simulink model "ADP_RPI"  (R2017a)
settings: Solver=FixedStepAuto  StartTime=0.0  StopTime=inf  RelTol=1e-3
InitFcn:
  | ADP_Init
  | RPI3_SPI_Int
values from neighbouring files (symbols this model uses):
  K = 0.5*(R_Mat_ADP^-1)*B'*P_Mat    [ADP_Init.m]
  T = 1    [ADP_Init.m]
  tau = 0.01    [ADP_Init.m]
  wcInit = weights    [ADP_Init.m]
undefined symbols (not defined in the file or in its folder): spiPeriod
libraries: simulink x4, embdlinuxlib x4, simulink_extras x2
settings Model: SimulationMode=external  ExtModeTrigDuration=10000  Creator=gjaniak  LastModifiedBy=gjaniak
settings SolverCC: PositivePriorityOrder=on
settings OptimizationCC: PassReuseOutputArgsAs=Individual arguments  MaxStackSize=64
settings DebuggingCC: ParameterTunabilityLossMsg=error
settings HardwareCC: ProdBitPerPointer=32  ProdBitPerSizeT=32  ProdBitPerPtrDiffT=32  ProdLargestAtomicInteger=Long  ProdLargestAtomicFloat=Double  ProdWordSize=32  ProdHWDeviceType=ARM Compatible->ARM Cortex
settings SFSimCC: MATLABDynamicMemAlloc=off
settings RTWCC: SystemTargetFile=ert.tlc  HardwareBoard=Raspberry Pi  TLCOptions="-aInlineSetEventsForThisBaseRateFcn=TLC_FALSE -aSuppressMultiTaskScheduler=TLC_FALSE  -aRateBasedStepFcn=0"  TemplateMakefile=ert_default_tmf  Description=Embedded Coder  GenerateReport=on  Toolchain=GNU GCC Raspberry Pi  IncludeHyperlinkInReport=on  LaunchReport=on  GenerateTraceInfo=on  GenerateTraceReport=on  GenerateTraceReportSl=on  GenerateTraceReportSf=on  GenerateTraceReportEml=on
settings CodeAppCC: ForceParamTrailComments=on  IgnoreCustomStorageClasses=off  OperatorAnnotations=on  SimulinkDataObjDesc=on  SFDataObjDesc=on  MATLABFcnDesc=on  InsertBlockDesc=on  MATLABSourceComments=on
settings ERTTargetCC: SupportContinuousTime=on  SupportVariableSizeSignals=on

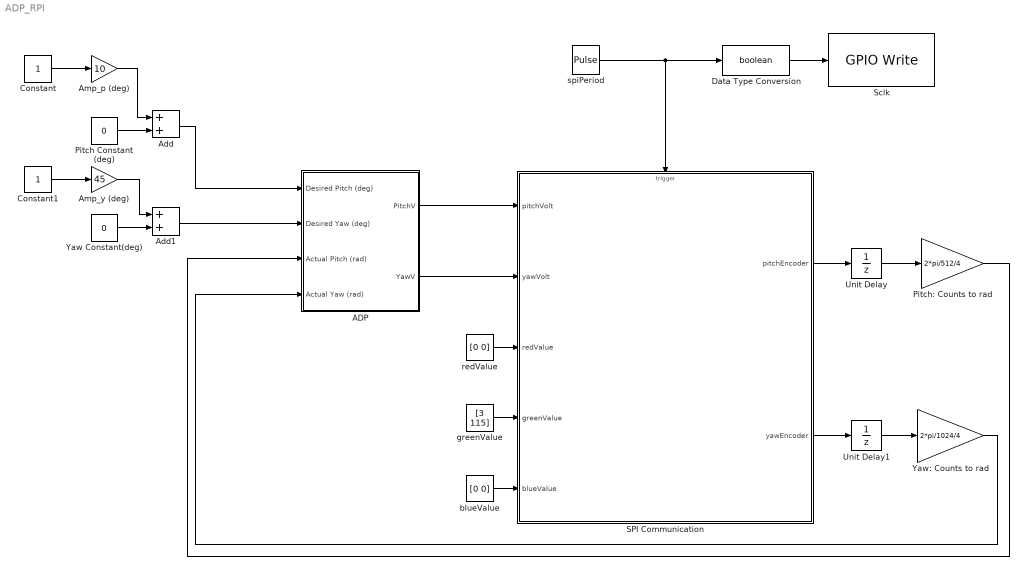
== system ADP_RPI ==
  ADP : Subsystem
  Add : Sum
  Add1 : Sum
  Amp_p (deg) : Gain  Gain=10
  Amp_y (deg) : Gain  Gain=45
  Constant : Constant
  Constant1 : Constant
  Data Type Conversion : DataTypeConversion  OutDataTypeStr=boolean
  Pitch Constant (deg) : Constant  Value=0
  Pitch: Counts to rad : Gain  Gain=2*pi/512/4
  SPI Communication : Subsystem  TreatAsAtomicUnit=on
  Sclk : embdlinuxlib/GPIO Write  board=Pi 3 Model B  gpio=11  direction=Output  blockPlatform=Raspberry Pi
  Unit Delay : UnitDelay  SampleTime=-1
  Unit Delay1 : UnitDelay  SampleTime=-1
  Yaw Constant(deg) : Constant  Value=0
  Yaw: Counts to rad : Gain  Gain=2*pi/1024/4
  blueValue : Constant  Value=[0 0]
  greenValue : Constant  Value=[3 115]
  redValue : Constant  Value=[0 0]
  spiPeriod : DiscretePulseGenerator  PulseType=Time based  Period=spiPeriod  PulseWidth=50
  wires:
  Pitch Constant (deg)/1 -> Add/2
  Amp_p (deg)/1 -> Add/1
  Yaw Constant(deg)/1 -> Add1/2
  Amp_y (deg)/1 -> Add1/1
  Constant/1 -> Amp_p (deg)/1
  Constant1/1 -> Amp_y (deg)/1
  Data Type Conversion/1 -> Sclk/1
  blueValue/1 -> SPI Communication/5(blueValue)
  Unit Delay1/1 -> Yaw: Counts to rad/1
  spiPeriod/1 -> SPI Communication/Trigger, Data Type Conversion/1
  SPI Communication/1(pitchEncoder) -> Unit Delay/1
  SPI Communication/2(yawEncoder) -> Unit Delay1/1
  greenValue/1 -> SPI Communication/4(greenValue)
  redValue/1 -> SPI Communication/3(redValue)
  Unit Delay/1 -> Pitch: Counts to rad/1
  ADP/1(PitchV) -> SPI Communication/1(pitchVolt)
  ADP/2(YawV) -> SPI Communication/2(yawVolt)
  Add/1 -> ADP/1(Desired Pitch (deg))
  Add1/1 -> ADP/2(Desired Yaw (deg))
  Yaw: Counts to rad/1 -> ADP/4(Actual Yaw (rad))
  Pitch: Counts to rad/1 -> ADP/3(Actual Pitch (rad))

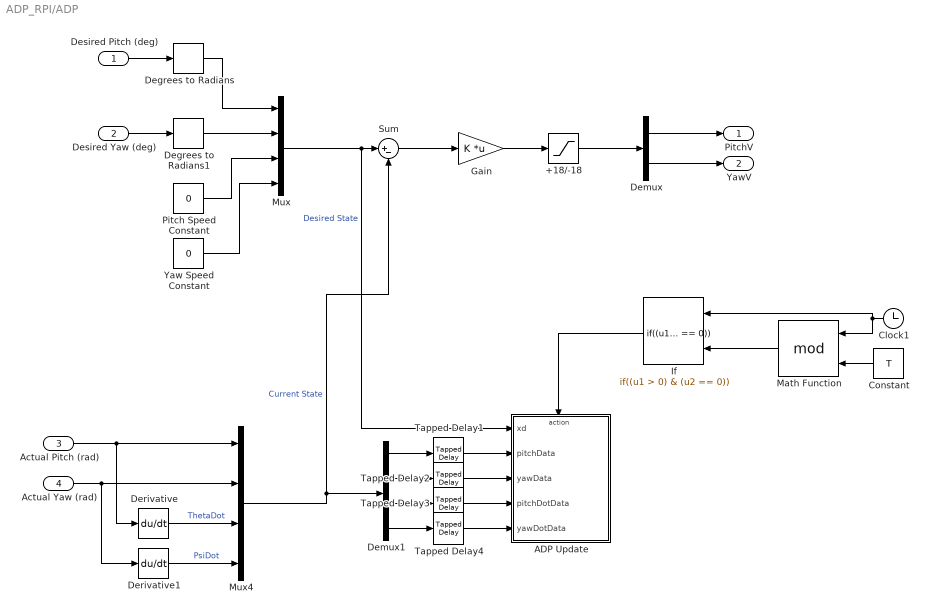
== system ADP_RPI/ADP ==
  Desired Pitch (deg) : Inport
  Desired Yaw (deg) : Inport  Port=2
  Actual Pitch (rad) : Inport  Port=3
  Actual Yaw (rad) : Inport  Port=4
  +18/-18 : Saturate  UpperLimit=18  LowerLimit=-18
  ADP Update : Subsystem  TreatAsAtomicUnit=on
  Clock1 : Clock
  Constant : Constant  Value=T
  Degrees to Radians : simulink_extras/Transformations/Degrees to Radians
  Degrees to Radians1 : simulink_extras/Transformations/Degrees to Radians
  Demux : Demux  Outputs=2
  Demux1 : Demux
  Derivative : Derivative
  Derivative1 : Derivative
  Gain : Gain  Gain=K  Multiplication=Matrix(K*u)
  If : If  NumInputs=2  IfExpression=(u1 > 0) & (u2 == 0)  ShowElse=off
  Math Function : Math  Operator=mod  SaturateOnIntegerOverflow=on
  Mux : Mux
  Mux4 : Mux
  Pitch Speed Constant : Constant  Value=0
  Sum : Sum  Inputs=|+-
  Tapped Delay{1..4} (4 alike) : simulink/Discrete/Tapped Delay  vinit=0.0  samptime=-1  NumDelays=floor(T/tau)  DelayOrder=Oldest  includeCurrent=off
  Yaw Speed Constant : Constant  Value=0
  PitchV : Outport
  YawV : Outport  Port=2
  wires:
  Sum/1 -> Gain/1
  Gain/1 -> +18/-18/1
  +18/-18/1 -> Demux/1
  Demux/1 -> PitchV/1
  Demux/2 -> YawV/1
  If/1 -> ADP Update/Action
  Math Function/1 -> If/2
  Constant/1 -> Math Function/2
  Clock1/1 -> If/1, Math Function/1
  Demux1/1 -> Tapped Delay1/1
  Tapped Delay1/1 -> ADP Update/2(pitchData)
  Demux1/2 -> Tapped Delay2/1
  Tapped Delay2/1 -> ADP Update/3(yawData)
  Demux1/3 -> Tapped Delay3/1
  Tapped Delay3/1 -> ADP Update/4(pitchDotData)
  Demux1/4 -> Tapped Delay4/1
  Tapped Delay4/1 -> ADP Update/5(yawDotData)
  Mux/1 -> ADP Update/1(xd), Sum/1  "Desired State"
  Degrees to Radians1/1 -> Mux/2
  Yaw Speed Constant/1 -> Mux/4
  Degrees to Radians/1 -> Mux/1
  Pitch Speed Constant/1 -> Mux/3
  Desired Pitch (deg)/1 -> Degrees to Radians/1
  Desired Yaw (deg)/1 -> Degrees to Radians1/1
  Actual Pitch (rad)/1 -> Mux4/1, Derivative/1
  Actual Yaw (rad)/1 -> Mux4/2, Derivative1/1
  Mux4/1 -> Sum/2, Demux1/1  "Current State"
  Derivative/1 -> Mux4/3  "ThetaDot"
  Derivative1/1 -> Mux4/4  "PsiDot"

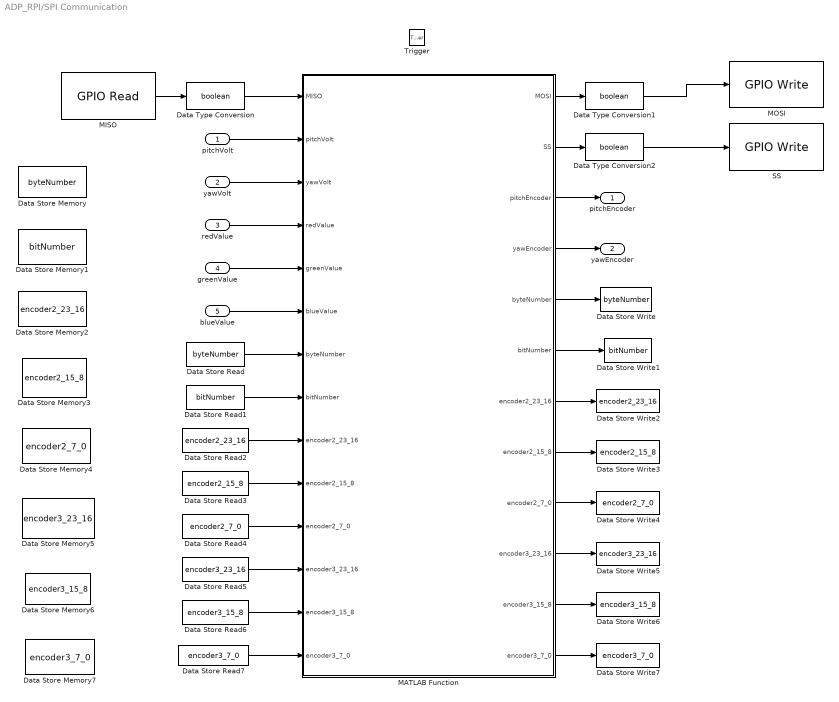
== system ADP_RPI/SPI Communication ==
  pitchVolt : Inport
  yawVolt : Inport  Port=2
  redValue : Inport  Port=3
  greenValue : Inport  Port=4
  blueValue : Inport  Port=5
  Trigger : TriggerPort  VariantControl=Variant
  Data Store Memory : DataStoreMemory  DataStoreName=byteNumber  ReadBeforeWriteMsg=warning  WriteAfterWriteMsg=warning  WriteAfterReadMsg=warning  ShowAdditionalParam=off
  Data Store Memory1 : DataStoreMemory  DataStoreName=bitNumber  ReadBeforeWriteMsg=warning  WriteAfterWriteMsg=warning  WriteAfterReadMsg=warning  ShowAdditionalParam=off
  Data Store Memory2 : DataStoreMemory  DataStoreName=encoder2_23_16  ReadBeforeWriteMsg=warning  WriteAfterWriteMsg=warning  WriteAfterReadMsg=warning  InitialValue=[0 0 0 0 0 0 0 0]  ShowAdditionalParam=off
  Data Store Memory3 : DataStoreMemory  DataStoreName=encoder2_15_8  ReadBeforeWriteMsg=warning  WriteAfterWriteMsg=warning  WriteAfterReadMsg=warning  InitialValue=[0 0 0 0 0 0 0 0]  ShowAdditionalParam=off
  Data Store Memory4 : DataStoreMemory  DataStoreName=encoder2_7_0  ReadBeforeWriteMsg=warning  WriteAfterWriteMsg=warning  WriteAfterReadMsg=warning  InitialValue=[0 0 0 0 0 0 0 0]  ShowAdditionalParam=off
  Data Store Memory5 : DataStoreMemory  DataStoreName=encoder3_23_16  ReadBeforeWriteMsg=warning  WriteAfterWriteMsg=warning  WriteAfterReadMsg=warning  InitialValue=[0 0 0 0 0 0 0 0]  ShowAdditionalParam=off
  Data Store Memory6 : DataStoreMemory  DataStoreName=encoder3_15_8  ReadBeforeWriteMsg=warning  WriteAfterWriteMsg=warning  WriteAfterReadMsg=warning  InitialValue=[0 0 0 0 0 0 0 0]  ShowAdditionalParam=off
  Data Store Memory7 : DataStoreMemory  DataStoreName=encoder3_7_0  ReadBeforeWriteMsg=warning  WriteAfterWriteMsg=warning  WriteAfterReadMsg=warning  InitialValue=[0 0 0 0 0 0 0 0]  ShowAdditionalParam=off
  Data Store Read1 : DataStoreRead  DataStoreName=bitNumber
  Data Store Read2 : DataStoreRead  DataStoreName=encoder2_23_16
  Data Store Read3 : DataStoreRead  DataStoreName=encoder2_15_8
  Data Store Read4 : DataStoreRead  DataStoreName=encoder2_7_0
  Data Store Read5 : DataStoreRead  DataStoreName=encoder3_23_16
  Data Store Read6 : DataStoreRead  DataStoreName=encoder3_15_8
  Data Store Read7 : DataStoreRead  DataStoreName=encoder3_7_0
  Data Store Write : DataStoreWrite  DataStoreName=byteNumber
  Data Store Write1 : DataStoreWrite  DataStoreName=bitNumber
  Data Store Write2 : DataStoreWrite  DataStoreName=encoder2_23_16
  Data Store Write3 : DataStoreWrite  DataStoreName=encoder2_15_8
  Data Store Write4 : DataStoreWrite  DataStoreName=encoder2_7_0
  Data Store Write5 : DataStoreWrite  DataStoreName=encoder3_23_16
  Data Store Write6 : DataStoreWrite  DataStoreName=encoder3_15_8
  Data Store Write7 : DataStoreWrite  DataStoreName=encoder3_7_0
  Data Store Read : DataStoreRead  DataStoreName=byteNumber
  Data Type Conversion : DataTypeConversion  OutDataTypeStr=boolean
  Data Type Conversion1 : DataTypeConversion  OutDataTypeStr=boolean
  Data Type Conversion2 : DataTypeConversion  OutDataTypeStr=boolean
  MATLAB Function : MATLAB Function  TreatAsAtomicUnit=on
  MISO : embdlinuxlib/GPIO Read  board=Pi 3 Model B  gpio=9  internalResistor=Off  sampleTime=inf  direction=Input  blockPlatform=Raspberry Pi
  MOSI : embdlinuxlib/GPIO Write  board=Pi 3 Model B  gpio=10  direction=Output  blockPlatform=Raspberry Pi
  "SS " : embdlinuxlib/GPIO Write  board=Pi 3 Model B  gpio=8  direction=Output  blockPlatform=Raspberry Pi
  pitchEncoder : Outport
  yawEncoder : Outport  Port=2
  wires:
  blueValue/1 -> MATLAB Function/6(blueValue)
  greenValue/1 -> MATLAB Function/5(greenValue)
  redValue/1 -> MATLAB Function/4(redValue)
  yawVolt/1 -> MATLAB Function/3(yawVolt)
  pitchVolt/1 -> MATLAB Function/2(pitchVolt)
  MATLAB Function/4(yawEncoder) -> yawEncoder/1
  MATLAB Function/3(pitchEncoder) -> pitchEncoder/1
  Data Type Conversion/1 -> MATLAB Function/1(MISO)
  MATLAB Function/1(MOSI) -> Data Type Conversion1/1
  MATLAB Function/2(SS) -> Data Type Conversion2/1
  MISO/1 -> Data Type Conversion/1
  Data Type Conversion1/1 -> MOSI/1
  Data Type Conversion2/1 -> "SS "/1
  Data Store Read/1 -> MATLAB Function/7("byteNumber ")
  Data Store Read1/1 -> MATLAB Function/8("bitNumber ")
  Data Store Read2/1 -> MATLAB Function/9("encoder2_23_16 ")
  Data Store Read3/1 -> MATLAB Function/10("encoder2_15_8 ")
  Data Store Read4/1 -> MATLAB Function/11("encoder2_7_0 ")
  Data Store Read5/1 -> MATLAB Function/12("encoder3_23_16 ")
  Data Store Read6/1 -> MATLAB Function/13("encoder3_15_8 ")
  Data Store Read7/1 -> MATLAB Function/14("encoder3_7_0 ")
  MATLAB Function/5(byteNumber) -> Data Store Write/1
  MATLAB Function/6(bitNumber) -> Data Store Write1/1
  MATLAB Function/7(encoder2_23_16) -> Data Store Write2/1
  MATLAB Function/8(encoder2_15_8) -> Data Store Write3/1
  MATLAB Function/9(encoder2_7_0) -> Data Store Write4/1
  MATLAB Function/10(encoder3_23_16) -> Data Store Write5/1
  MATLAB Function/11(encoder3_15_8) -> Data Store Write6/1
  MATLAB Function/12(encoder3_7_0) -> Data Store Write7/1

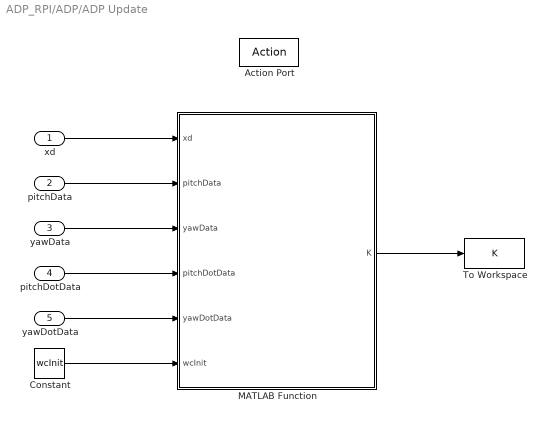
== system ADP_RPI/ADP/ADP Update ==
  xd : Inport
  pitchData : Inport  Port=2
  yawData : Inport  Port=3
  pitchDotData : Inport  Port=4
  yawDotData : Inport  Port=5
  Action Port : ActionPort  ActionType=then
  Constant : Constant  Value=wcInit
  MATLAB Function : MATLAB Function  TreatAsAtomicUnit=on
  To Workspace : ToWorkspace  VariableName=K  SampleTime=-1
  wires:
  MATLAB Function/1(K) -> To Workspace/1
  yawData/1 -> MATLAB Function/3(yawData)
  pitchDotData/1 -> MATLAB Function/4(pitchDotData)
  yawDotData/1 -> MATLAB Function/5(yawDotData)
  pitchData/1 -> MATLAB Function/2(pitchData)
  xd/1 -> MATLAB Function/1(xd)
  Constant/1 -> MATLAB Function/6(wcInit)

== matlab function ADP_RPI/SPI Communication/MATLAB Function ==
  data: MISO input; MOSI output; pitchVolt input; yawVolt input; redValue input; greenValue input; blueValue input; byteNumber input; bitNumber input; encoder2_23_16 input; encoder2_15_8 input; encoder2_7_0 input; encoder3_23_16 input; encoder3_15_8 input; encoder3_7_0 input; SS output; pitchEncoder output; yawEncoder output; byteNumber output; bitNumber output; encoder2_23_16 output; encoder2_15_8 output; encoder2_7_0 output; encoder3_23_16 output; encoder3_15_8 output; encoder3_7_0 output
% THIS FUNCTION CONTROLS THE SPI INTERFACING
% THIS FUNCTION DETERMINES WHAT DATA IS SENT TO THE QUANSER AERO AND WHAT
% DATA IS RETRIEVED FROM THE QUANSER AERO
function [MOSI,SS,pitchEncoder,yawEncoder,byteNumber,bitNumber,encoder2_23_16,encoder2_15_8,encoder2_7_0,encoder3_23_16,encoder3_15_8,encoder3_7_0] = fcn(MISO, pitchVolt,yawVolt,redValue,greenValue,blueValue,byteNumber,bitNumber,encoder2_23_16,encoder2_15_8,encoder2_7_0,encoder3_23_16,encoder3_15_8,encoder3_7_0)
% Variables used in the function
complement = '0000000000000000';
pitchEncoderBin = '000000000000000000000000';
yawEncoderBin = '000000000000000000000000';
tempBin = '00000000000000000000000000000000';
tempVoltBin = '00000000';

% Output the value of the pitch encoder using the latest byte values
% Combine all of the encoder bytes
pitchEncoderIn = [encoder2_23_16 encoder2_15_8 encoder2_7_0];
% Convert the encoder binary vector into a character array
for i = 1:24
    if (pitchEncoderIn(i) == 1)
        pitchEncoderBin(i) = '1';
    else
        pitchEncoderBin(i) = '0';
    end
end
% Calculate the 2's complement value of the encoder
if(pitchEncoderBin(1) == '1')
    for i = 1:32
        if (i < 9)
            tempBin(i) = '1';
        else
            tempBin(i) = pitchEncoderBin(i - 8);
        end
    end
else
    for i = 1:32
        if (i < 9)
            tempBin(i) = '0';
        else
            tempBin(i) = pitchEncoderBin(i - 8);
        end
    end
end
pitchEncoderTemp = typecast(uint32(bin2dec(tempBin)),'int32');
pitchEncoderOut = cast(pitchEncoderTemp,'double');
pitchEncoder = pitchEncoderOut(1);

% Output the value of the yaw encoder using the latest byte values
% Combine all of the encoder bytes
yawEncoderIn = [encoder3_23_16 encoder3_15_8 encoder3_7_0];
% Convert the encoder binary vector into a character array
for i = 1:24
    if (yawEncoderIn(i) == 1)
        yawEncoderBin(i) = '1';
    else
        yawEncoderBin(i) = '0';
    end
end
% Calculate the 2's complement value of the encoder
if(yawEncoderBin(1) == '1')
    for i = 1:32
        if (i < 9)
            tempBin(i) = '1';
        else
            tempBin(i) = yawEncoderBin(i - 8);
        end
    end
else
    for i = 1:32
        if (i < 9)
            tempBin(i) = '0';
        else
            tempBin(i) = yawEncoderBin(i - 8);
        end
    end
end
yawEncoderTemp = typecast(uint32(bin2dec(tempBin)),'int32');
yawEncoderOut = cast(yawEncoderTemp,'double');
yawEncoder = yawEncoderOut(1);

% Determine which byte we are currently sending
% Specify the slave select value
% - 0 to activate the SPI on the Quanser AERO
% - 1 to de-activate the SPI on the Quanser AERO
% Determine the what the byte to be transmitted should be
switch byteNumber
    case 0
    % ** START OF BASE PACKET **
    % BYTE 0
    % MOSI DATA - BASE MODE (0X01)
    % MISO DATA - BASE ID MSB
    % Beginning of the transmission, so SS goes low
    SS = 0;
    readyMOSI = dec2bin(1,8);        

    case 1
    % BYTE 1
    % MOSI DATA - PADDING BYTE (0X00)
    % MISO DATA - BASE ID LSB
    SS = 0;
    readyMOSI = dec2bin(0,8);

    case 2
    % BYTE 2
    % MOSI DATA - BASE WRITE MASK
    % MISO DATA - ENCODER 2 (23-16)
    SS = 0;
    % Enable the overwriting of encoders 2 and 3 and the LED colors
    % Bit 4 - Set encoder 3 enable
    % Bit 3 - Set encoder 2 enable
    % Bit 2 - Write blue LED
    % Bit 1 - Write green LED
    % Bit 0 - Write red LED
    % Don't want to overwrite the encoder values
    readyMOSI = dec2bin(7,8);
    % Receive the MISO byte bit by bit and update the vector holding the
    % byte
    switch bitNumber
        case 1
            if (MISO == true)
                encoder2_23_16(1) = 1;
            else
                encoder2_23_16(1) = 0;
            end
        case 2
            if (MISO == true)
                encoder2_23_16(2) = 1;
            else
                encoder2_23_16(2) = 0;
            end
        case 3
            if (MISO == true)
                encoder2_23_16(3) = 1;
            else
                encoder2_23_16(3) = 0;
            end
        case 4
            if (MISO == true)
                encoder2_23_16(4) = 1;
            else
                encoder2_23_16(4) = 0;
            end
        case 5
            if (MISO == true)
                encoder2_23_16(5) = 1;
            else
                encoder2_23_16(5) = 0;
            end
        case 6
            if (MISO == true)
                encoder2_23_16(6) = 1;
            else
                encoder2_23_16(6) = 0;
            end
        case 7
            if (MISO == true)
                encoder2_23_16(7) = 1;
            else
                encoder2_23_16(7) = 0;
            end
        case 8
            if (MISO == true)
                encoder2_23_16(8) = 1;
            else
                encoder2_23_16(8) = 0;
            end
    end
    
    case 3
    % BYTE 3
    % MOSI DATA - RED LED MSB
    % MISO DATA - ENCODER 2 (15-8)
    SS = 0;
    readyMOSI = dec2bin(redValue(1),8);
    % Receive the MISO byte bit by bit and update the vector holding the
    % byte
    switch bitNumber
        case 1
            if (MISO == true)
                encoder2_15_8(1) = 1;
            else
                encoder2_15_8(1) = 0;
            end
        case 2
            if (MISO == true)
                encoder2_15_8(2) = 1;
            else
                encoder2_15_8(2) = 0;
            end
        case 3
            if (MISO == true)
                encoder2_15_8(3) = 1;
            else
                encoder2_15_8(3) = 0;
            end
        case 4
            if (MISO == true)
                encoder2_15_8(4) = 1;
            else
                encoder2_15_8(4) = 0;
            end
        case 5
            if (MISO == true)
                encoder2_15_8(5) = 1;
            else
                encoder2_15_8(5) = 0;
            end
        case 6
            if (MISO == true)
                encoder2_15_8(6) = 1;
            else
                encoder2_15_8(6) = 0;
            end
        case 7
            if (MISO == true)
                encoder2_15_8(7) = 1;
            else
                encoder2_15_8(7) = 0;
            end
        case 8
            if (MISO == true)
                encoder2_15_8(8) = 1;
            else
                encoder2_15_8(8) = 0;
            end
    end

    case 4
    % BYTE 4
    % MOSI DATA - RED LED LSB
    % MISO DATA - ENCODER 2 (7-0)
    SS = 0;
    readyMOSI = dec2bin(redValue(2),8);
    % Receive the MISO byte bit by bit and update the vector holding the
    % byte
    switch bitNumber
        case 1
            if (MISO == true)
                encoder2_7_0(1) = 1;
            else
                encoder2_7_0(1) = 0;
            end
        case 2
            if (MISO == true)
                encoder2_7_0(2) = 1;
            else
                encoder2_7_0(2) = 0;
            end
        case 3
            if (MISO == true)
                encoder2_7_0(3) = 1;
            else
                encoder2_7_0(3) = 0;
            end
        case 4
            if (MISO == true)
                encoder2_7_0(4) = 1;
            else
                encoder2_7_0(4) = 0;
            end
        case 5
            if (MISO == true)
                encoder2_7_0(5) = 1;
            else
                encoder2_7_0(5) = 0;
            end
        case 6
            if (MISO == true)
                encoder2_7_0(6) = 1;
            else
                encoder2_7_0(6) = 0;
            end
        case 7
            if (MISO == true)
                encoder2_7_0(7) = 1;
            else
                encoder2_7_0(7) = 0;
            end
        case 8
            if (MISO == true)
                encoder2_7_0(8) = 1;
            else
                encoder2_7_0(8) = 0;
            end
    end

    case 5
    % BYTE 5
    % MOSI DATA - GREEN LED MSB
    % MISO DATA - ENCODER 3 (23-16)
    SS = 0;
    readyMOSI = dec2bin(greenValue(1),8);
    % Receive the MISO byte bit by bit and update the vector holding the
    % byte
    switch bitNumber
        case 1
            if (MISO == true)
                encoder3_23_16(1) = 1;
            else
                encoder3_23_16(1) = 0;
            end
        case 2
            if (MISO == true)
                encoder3_23_16(2) = 1;
            else
                encoder3_23_16(2) = 0;
            end
        case 3
            if (MISO == true)
                encoder3_23_16(3) = 1;
            else
                encoder3_23_16(3) = 0;
            end
        case 4
            if (MISO == true)
                encoder3_23_16(4) = 1;
            else
                encoder3_23_16(4) = 0;
            end
        case 5
            if (MISO == true)
                encoder3_23_16(5) = 1;
            else
                encoder3_23_16(5) = 0;
            end
        case 6
            if (MISO == true)
                encoder3_23_16(6) = 1;
            else
                encoder3_23_16(6) = 0;
            end
        case 7
            if (MISO == true)
                encoder3_23_16(7) = 1;
            else
                encoder3_23_16(7) = 0;
            end
        case 8
            if (MISO == true)
                encoder3_23_16(8) = 1;
            else
                encoder3_23_16(8) = 0;
            end
    end

    case 6
    % BYTE 6
    % MOSI DATA - GREEN LED LSB
    % MISO DATA - ENCODER 3 (15-8)
    SS = 0;
    readyMOSI = dec2bin(greenValue(2),8);
    % Receive the MISO byte bit by bit and update the vector holding the
    % byte
    switch bitNumber
        case 1
            if (MISO == true)
                encoder3_15_8(1) = 1;
            else
                encoder3_15_8(1) = 0;
            end
        case 2
            if (MISO == true)
                encoder3_15_8(2) = 1;
            else
                encoder3_15_8(2) = 0;
            end
        case 3
            if (MISO == true)
                encoder3_15_8(3) = 1;
            else
                encoder3_15_8(3) = 0;
            end
        case 4
            if (MISO == true)
                encoder3_15_8(4) = 1;
            else
                encoder3_15_8(4) = 0;
            end
        case 5
            if (MISO == true)
                encoder3_15_8(5) = 1;
            else
                encoder3_15_8(5) = 0;
            end
        case 6
            if (MISO == true)
                encoder3_15_8(6) = 1;
            else
                encoder3_15_8(6) = 0;
            end
        case 7
            if (MISO == true)
                encoder3_15_8(7) = 1;
            else
                encoder3_15_8(7) = 0;
            end
        case 8
            if (MISO == true)
                encoder3_15_8(8) = 1;
            else
                encoder3_15_8(8) = 0;
            end
    end

    case 7
    % BYTE 7
    % MOSI DATA - BLUE LED MSB
    % MISO DATA - ENCODER 3 (7-0)
    SS = 0;
    readyMOSI = dec2bin(blueValue(1),8);
    % Receive the MISO byte bit by bit and update the vector holding the
    % byte
    switch bitNumber
        case 1
            if (MISO == true)
                encoder3_7_0(1) = 1;
            else
                encoder3_7_0(1) = 0;
            end
        case 2
            if (MISO == true)
                encoder3_7_0(2) = 1;
            else
                encoder3_7_0(2) = 0;
            end
        case 3
            if (MISO == true)
                encoder3_7_0(3) = 1;
            else
                encoder3_7_0(3) = 0;
            end
        case 4
            if (MISO == true)
                encoder3_7_0(4) = 1;
            else
                encoder3_7_0(4) = 0;
            end
        case 5
            if (MISO == true)
                encoder3_7_0(5) = 1;
            else
                encoder3_7_0(5) = 0;
            end
        case 6
            if (MISO == true)
                encoder3_7_0(6) = 1;
            else
                encoder3_7_0(6) = 0;
            end
        case 7
            if (MISO == true)
                encoder3_7_0(7) = 1;
            else
                encoder3_7_0(7) = 0;
            end
        case 8
            if (MISO == true)
                encoder3_7_0(8) = 1;
            else
                encoder3_7_0(8) = 0;
            end
    end

    case 8
    % BYTE 8
    % MOSI DATA - BLUE LED LSB
    % MISO DATA - TACHOMETER 2 (23-16)
    SS = 0;
    readyMOSI = dec2bin(blueValue(2),8);

    case 9
    % BYTE 9
    % MOSI DATA - SET ENCODER 2 (23-16)
    % MISO DATA - TACHOMETER 2 (15-8)
    SS = 0;
    readyMOSI = dec2bin(0,8);

    case 10
    % BYTE 10
    % MOSI DATA - SET ENCODER 2 (15-8)
    % MISO DATA - TACHOMETER 2 (7-0)
    SS = 0;
    readyMOSI = dec2bin(0,8);

    case 11
    % BYTE 11
    % MOSI DATA - SET ENCODER 2 (7-0)
    % MISO DATA - TACHOMETER 3 (23-16)
    SS = 0;
    readyMOSI = dec2bin(0,8);

    case 12
    % BYTE 12
    % MOSI DATA - SET ENCODER 3 (23-16)
    % MISO DATA - TACHOMETER 3 (15-8)
    SS = 0;
    readyMOSI = dec2bin(0,8);

    case 13
    % BYTE 13
    % MOSI DATA - SET ENCODER 3 (15-8)
    % MISO DATA - TACHOMETER 3 (7-0)
    SS = 0;
    readyMOSI = dec2bin(0,8);

    case 14
    % BYTE 14
    % MOSI DATA - SET ENCODER 3 (7-0)
    % MISO DATA - RESERVED (0X00)
    SS = 0;
    readyMOSI = dec2bin(0,8);
    
    case 15
    % ** START OF CORE PACKET **
    % BYTE 15
    % MOSI DATA - CORE MODE (0X01)
    % MISO DATA - CORE ID MSB
    SS = 0;
    readyMOSI = dec2bin(1,8);

    case 16
    % BYTE 16
    % MOSI DATA - PADDING BYTE (0X00)
    % MISO DATA - CORE ID LSB
    SS = 0;
    readyMOSI = dec2bin(0,8);

    case 17
    % BYTE 17
    % MOSI DATA - CORE WRITE MASK
    % MISO DATA - CURRENT SENSE 0 (15-8)
    SS = 0;
    % Do not enable the overwriting of encoders 0 and 1, but do enable the
    % overwriting of the motor voltages
    % Bit 5 - Set encoder 1 enable
    % Bit 4 - Set encoder 0 enable
    % Bit 3 - Write motor 1 voltage
    % Bit 2 - Write motor 1 enable
    % Bit 1 - Write motor 0 voltage
    % Bit 0 - Write motor 0 enable
    readyMOSI = dec2bin(15,8);

    case 18
    % BYTE 18
    % MOSI DATA - MOTOR 0 COMMAND (15-8)
    % MISO DATA - CURRENT SENSE 0 (7-0)
    SS = 0;
    % Convert the desired voltage to a value between -999 and 999
    % 24 is the saturation level in the model
    pitchVoltTemp = ceil((999*pitchVolt)/24);
    % If the desired voltage is positive, concatenate a '1' to the front of
    % the voltage value
    % Pass the MSB of the new value
    if (sign(pitchVoltTemp) == 1)
        temp = dec2bin(pitchVoltTemp,15);
        for i = 1:8
            if (i == 1)
                tempVoltBin(i) = '1';
            else
                tempVoltBin(i) = temp(i - 1);
            end
        end
        readyMOSI = tempVoltBin;
    % If the desired voltage is negative, find the 2's complement value of
    % the voltage
    elseif (sign(pitchVoltTemp) == -1)
        temp = dec2bin(-1*pitchVoltTemp,15);
        % Find the complement
        for i = 1:15
            if (temp(i) == '1')
                complement(i) = '0';
            else
                complement(i) = '1';
            end
        end
        temp1 = bin2dec(complement) + 1;
        temp2 = dec2bin(temp1,15);
        for i = 1:8
            if (i == 1)
                tempVoltBin(i) = '1';
            else
                tempVoltBin(i) = temp2(i - 1);
            end
        end
        readyMOSI = tempVoltBin;
    % If the desired voltage is zero, don't activate the motor
    else
        readyMOSI = dec2bin(0,8);
    end

    case 19
    % BYTE 19
    % MOSI DATA - MOTOR 0 COMMAND (7-0)
    % MISO DATA - CURRENT SENSE 1 (15-8)
    SS = 0;
    % Convert the desired voltage to a value between -999 and 999
    % 24 is the saturation level in the model
    pitchVoltTemp = ceil((999*pitchVolt)/24);
    % If the voltage is positive, pass the LSB
    if (sign(pitchVoltTemp) == 1)
        temp = dec2bin(pitchVoltTemp,15);
        readyMOSI = temp(8:15);
    % If the voltage is negative, find the 2's complement value and then
    % pass the LSB
    elseif (sign(pitchVoltTemp) == -1)
        temp = dec2bin(-1*pitchVoltTemp,15);
        % Find the complement
        for i = 1:15
            if (temp(i) == '1')
                complement(i) = '0';
            else
                complement(i) = '1';
            end
        end
        temp1 = bin2dec(complement) + 1;
        temp2 = dec2bin(temp1,15);
        readyMOSI = temp2(8:15);
    % If the desired voltage is zero, do not activate the motor
    else
        readyMOSI = dec2bin(0,8);
    end

    case 20
    % BYTE 20
    % MOSI DATA - MOTOR 1 COMMAND (15-8)
    % MISO DATA - CURRENT SENSE 1 (7-0)
    SS = 0;
     % Convert the desired voltage to a value between -999 and 999
    % 24 is the saturation level in the model
    yawVoltTemp = ceil((999*yawVolt)/24);
    % If the desired voltage is positive, concatenate a '1' to the front of
    % the voltage value
    % Pass the MSB of the new value
    if (sign(yawVoltTemp) == 1)
        temp = dec2bin(yawVoltTemp,15);
        for i = 1:8
            if (i == 1)
                tempVoltBin(i) = '1';
            else
                tempVoltBin(i) = temp(i - 1);
            end
        end
        readyMOSI = tempVoltBin;
    % If the desired voltage is negative, find the 2's complement value of
    % the voltage
    elseif (sign(yawVoltTemp) == -1)
        temp = dec2bin(-1*yawVoltTemp,15);
        % Find the complement
        for i = 1:15
            if (temp(i) == '1')
                complement(i) = '0';
            else
                complement(i) = '1';
            end
        end
        temp1 = bin2dec(complement) + 1;
        temp2 = dec2bin(temp1,15);
        for i = 1:8
            if (i == 1)
                tempVoltBin(i) = '1';
            else
                tempVoltBin(i) = temp2(i - 1);
            end
        end
        readyMOSI = tempVoltBin;
    % If the desired voltage is zero, don't activate the motor
    else
        readyMOSI = dec2bin(0,8);
    end

    case 21
    % BYTE 21
    % MOSI DATA - MOTOR 1 COMMAND (7-0)
    % MISO DATA - TACHOMETER 0 (23-16)
    SS = 0;
    % Convert the desired voltage to a value between -999 and 999
    % 24 is the saturation level in the model
    yawVoltTemp = ceil((999*yawVolt)/24);
    % If the voltage is positive, pass the LSB
    if (sign(yawVoltTemp) == 1)
        temp = dec2bin(yawVoltTemp,15);
        readyMOSI = temp(8:15);
    % If the voltage is negative, find the 2's complement value and then
    % pass the LSB
    elseif (sign(yawVoltTemp) == -1)
        temp = dec2bin(-1*yawVoltTemp,15);
        for i = 1:15
            if (temp(i) == '1')
                complement(i) = '0';
            else
                complement(i) = '1';
            end
        end
        temp1 = bin2dec(complement) + 1;
        temp2 = dec2bin(temp1,15);
        readyMOSI = temp2(8:15);
    % If the desired voltage is zero, do not activate the motor
    else
        readyMOSI = dec2bin(0,8);
    end

    case 22
    % BYTE 22
    % MOSI DATA - SET ENCODER 0 (23-16)
    % MISO DATA - TACHOMETER 0 (15-8)
    SS = 0;
    readyMOSI = dec2bin(0,8);

    case 23
    % BYTE 23
    % MOSI DATA - SET ENCODER (7-0)
    % MISO DATA - TACHOMETER 0 (7-0)
    SS = 0;
    readyMOSI = dec2bin(0,8);

    case 24
    % BYTE 24
    % MOSI DATA - SET ENCODER 0 (7-0)
    % MISO DATA - TACHOMETER 1 (23-16)
    SS = 0;
    readyMOSI = dec2bin(0,8);

    case 25
    % BYTE 25
    % MOSI DATA - SET ENCODER 1 (23-16)
    % MISO DATA - TACHOMETER 1 (15-8)
    SS = 0;
    readyMOSI = dec2bin(0,8);

    case 26
    % BYTE 26
    % MOSI DATA - SET ENCODER 1 (15-8)
    % MISO DATA - TACHOMETER 1 (7-0)
    SS = 0;
    readyMOSI = dec2bin(0,8);

    case 27
    % BYTE 27
    % MOSI DATA - SET ENCODER 1 (7-0)
    % MISO DATA - STATUS
    SS = 0;
    readyMOSI = dec2bin(0,8);

    case 28
    % BYTE 28
    % MOSI DATA - PADDING BYTE (0X00)
    % MISO DATA - ENCODER 0 (23-16)
    SS = 0;
    readyMOSI = dec2bin(0,8);

    case 29
    % BYTE 29
    % MOSI DATA - PADDING BYTE (0X00)
    % MISO DATA - ENCODER 0 (15-8)
    SS = 0;
    readyMOSI = dec2bin(0,8);

    case 30
    % BYTE 30
    % MOSI DATA - PADDING BYTE (0X00)
    % MISO DATA - ENCODER 0 (7-0)
    SS = 0;
    readyMOSI = dec2bin(0,8);

    case 31
    % BYTE 31
    % MOSI DATA - PADDING BYTE (0X00)
    % MISO DATA - ENCODER 1 (23-16)
    SS = 0;
    readyMOSI = dec2bin(0,8);
    
    case 32
    % BYTE 32
    % MOSI DATA - PADDING BYTE (0X00)
    % MISO DATA - ENCODER 1 (15-8)
    SS = 0;
    readyMOSI = dec2bin(0,8);

    case 33
    % BYTE 33
    % MOSI DATA - PADDING BYTE (0X00)
    % MISO DATA - ENCODER 1 (7-0)
    SS = 0;
    readyMOSI = dec2bin(0,8);

    case 34
    % BYTE 34
    % MOSI DATA - PADDING BYTE (0X00)
    % MISO DATA - ACCELEROMETER X (15-8)
    SS = 0;
    readyMOSI = dec2bin(0,8);
    
    case 35
    % BYTE 35
    % MOSI DATA - PADDING BYTE (0X00)
    % MISO DATA - ACCELEROMETER X (7-0)
    SS = 0;
    readyMOSI = dec2bin(0,8);

    case 36
    % BYTE 36
    % MOSI DATA - PADDING BYTE (0X00)
    % MISO DATA - ACCELEROMETER Y (15-8)
    SS = 0;
    readyMOSI = dec2bin(0,8);

    case 37
    % BYTE 37
    % MOSI DATA - PADDING BYTE (0X00)
    % MISO DATA - ACCELEROMETER Y (7-0)
    SS = 0;
    readyMOSI = dec2bin(0,8);

    case 38
    % BYTE 38
    % MOSI DATA - PADDING BYTE (0X00)
    % MISO DATA - ACCELEROMETER Z (15-8)
    SS = 0;
    readyMOSI = dec2bin(0,8);

    case 39
    % BYTE 39
    % MOSI DATA - PADDING BYTE (0X00)
    % MISO DATA - ACCELEROMETER Z (7-0)
    SS = 0;
    readyMOSI = dec2bin(0,8);

    case 40
    % BYTE 40
    % MOSI DATA - PADDING BYTE (0X00)
    % MISO DATA - GYROSCOPE X (15-8)
    SS = 0;
    readyMOSI = dec2bin(0,8);

    case 41
    % BYTE 41
    % MOSI DATA - PADDING BYTE (0X00)
    % MISO DATA - GYROSCOPE X (7-0)
    SS = 0;
    readyMOSI = dec2bin(0,8);

    case 42
    % BYTE 42
    % MOSI DATA - PADDING BYTE (0X00)
    % MISO DATA - GYROSCOPE Y (15-8)
    SS = 0;
    readyMOSI = dec2bin(0,8);

    case 43
    % BYTE 43
    % MOSI DATA - PADDING BYTE (0X00)
    % MISO DATA - GYROSCOPE Y (7-0)
    SS = 0;
    readyMOSI = dec2bin(0,8);

    case 44
    % BYTE 44
    % MOSI DATA - PADDING BYTE (0X00)
    % MISO DATA - GYROSCOPE Z (15-8)
    SS = 0;
    readyMOSI = dec2bin(0,8);

    case 45
    % BYTE 45
    % MOSI DATA - PADDING BYTE (0X00)
    % MISO DATA - GYROSCOPE Z (7-0)
    SS = 0;
    readyMOSI = dec2bin(0,8);

    case 46
    % BYTE 46
    % MOSI DATA - PADDING BYTE (0X00)
    % MISO DATA - RESERVED (0X00)
    SS = 0;
    readyMOSI = dec2bin(0,8);

    case 47
    % BYTE 47
    % MOSI DATA - PADDING BYTE (0X00)
    % MISO DATA - RESERVED (0X00)
    SS = 0;
    readyMOSI = dec2bin(0,8);

    case 48
    % BYTE 48
    % MOSI DATA - PADDING BYTE (0X00)
    % MISO DATA - RESERVED (0X00)
    SS = 0;
    readyMOSI = dec2bin(0,8);

    case 49
    % BYTE 49
    % MOSI DATA - PADDING BYTE (0X00)
    % MISO DATA - RESERVED (0X00)
    SS = 0;
    readyMOSI = dec2bin(0,8);

    case 50
    % BYTE 50
    % MOSI DATA - PADDING BYTE (0X00)
    % MISO DATA - RESERVED (0X00)
    readyMOSI = dec2bin(0,8);
    % Reset the the slave select to begin the process again
    % Maybe not needed
    SS = 1;
    
    otherwise
    % Just in case
    readyMOSI = dec2bin(0,8);
    SS = 0;
end
% Pass the byte we have derived bit by bit
% Use the character array to determine the bit value
switch bitNumber
    case 1
        if (readyMOSI(1) == '1')
            MOSI = 1;
        else
            MOSI = 0;
        end
    case 2
        if (readyMOSI(2) == '1')
            MOSI = 1;
        else
            MOSI = 0;
        end
    case 3
        if (readyMOSI(3) == '1')
            MOSI = 1;
        else
            MOSI = 0;
        end
    case 4
        if (readyMOSI(4) == '1')
            MOSI = 1;
        else
            MOSI = 0;
        end
    case 5
        if (readyMOSI(5) == '1')
            MOSI = 1;
        else
            MOSI = 0;
        end
    case 6
        if (readyMOSI(6) == '1')
            MOSI = 1;
        else
            MOSI = 0;
        end
    case 7
        if (readyMOSI(7) == '1')
            MOSI = 1;
        else
            MOSI = 0;
        end
    case 8
        if (readyMOSI(8) == '1')
            MOSI = 1;
        else
            MOSI = 0;
        end
        % If we have just sent the last bit, update the byte number
        byteNumber = byteNumber + 1;
        % Reset back to zero if we have finished one transfer
        if (byteNumber == 51)
            byteNumber = 0;
        end
    otherwise
        MOSI = 0;
end
% Update the bit number that we are sending
bitNumber = bitNumber + 1;
% Reset back to 1 if we have finished one byte
if (bitNumber == 9)
    bitNumber = 1;
end
end

== matlab function ADP_RPI/ADP/ADP Update/MATLAB Function ==
  data: xd input; pitchData input; yawData input; pitchDotData input; yawDotData input; K output; wcInit input
% CRITIC WEIGHT TUNING NEURAL NETWORK
% This function is specific to the helicopter because of the number of
% weights and error model
% THIS FUNCTION CANNOT HAVE ANY ANONYMOUS FUNCTIONS DUE TO THE C CODE
% GENERATION UNSUPPORTING IT
function K = quanserAEROCriticTuning(xd,pitchData,yawData,pitchDotData,yawDotData,wcInit)
    % CREATE THE ERROR VECTOR MATRIX
    % Use the data from the tapped delay blocks to create the error state
    % vector matrix
    e_vec = [pitchData'; yawData'; pitchDotData'; yawDotData'];
    
    % REFERENCE DR. MIAH'S PAPER FOR EQUATION NUMBERS
    % Sampling time [s]
    tau = 0.05;
    
    % COST FUNCTION
    % Q and R matrices used in the cost function
    Q_Mat = diag([270 100 1 1]);
    R_Mat = 0.005*diag([1 1]);
    
    % SYSTEM PARAMETERS SPECIFIC TO THE 2-DOF QUANSER AERO
    A = [0 0 1 0; 0 0 0 1; -1.7442 0 -0.3307 0; 0 0 0 -0.9283];
    B = [0 0; 0 0; -0.0149 0.0414; -0.0751 -0.1295];
    % UNCOMMENT TO USE A STATE-SPACE MODEL THAT IS NOT THE CORRECT ONE DERIVED
    % A = [1 1 1 1; 1 1 1 1; 1 1 1 1; 1 1 1 1];
    % B = [0 0; 0 0; 0.1 0.1; -0.3 -0.3];
    % System dimensions specific for our model
    [n,~] = size(B);
    
    % ERROR MODEL OF THE HELICOPTER
    % gbar and hbar -- EQ 8
    % An anonymous function cannot be used for fbar
    gbar = -B;
    hbar = -A*xd;
    
    % DISCRETE-TIME ERROR MODEL FOR TIME TAU
    % g and h -- EQ 10
    % An anonymous function cannot be used for f
    g = gbar*tau;
    h = hbar*tau;
    
    % COST FUNCTION PARAMETERS
    % The Q matrix cannot be treated as an anonymous function as in the
    % MATLAB simulations
    % Control penalizing matrix in the continuous cost function
    Rbar = R_Mat;
    % The discrete-time cost function will have terms:
    % Right after EQ 11 in paper
    % Control penalizing matrix in the discretized cost function
    R = Rbar*tau;
    
    % NEURAL NETWORK FUNCTIONS
    % These functions cannot be written as anonymous functions as in the
    % MATLAB simulations
    
    % TOLERANCES
    % Convergence tolerance for control policy 
    EpsilonPolicy = 0.1;
    % Convergence tolerance for critic neural network
    EpsilonWcritic = 0.1;
    
    % TRAINING PARAMETERS
    % Number of outer loop iterations
    outerLoopMax = 700;
    % Number of inner loop iterations
    innerLoopMax = 100;
    % Number of equations needed for training, number of sub-intervals
    % Number of training samples
    [~,nbar] = size(e_vec);

    % WEIGHT INITIALIZATION
    % Initialize the weights of the critic neural network to zero
    % Number of rows hard-coded for the helicopter
    WcLast = zeros(14,1);
    
    % LEAST-SQUARES COMPUTATION INITIALIZATION
    % Matrices required for computing least squares weights of the critic 
    % neural networks -- EQ 20
    V = zeros(nbar,1);
    Lambda = zeros(nbar,14);
    
    % Matrix to hold the derivative of the error model during policy
    % updating
    e_k_plus_1 = zeros(n,nbar);
    
    % Product of the least squares matrices must be invertible
    % Logic flag indicating if the critic weights are unsolvable
    % The weights are unsolvable because the least squares matrices have no
    % solution -- not invertible
    diverged = 0;
    
    % OUTER LOOP
    for i = 1:(outerLoopMax-1)
    % Determine if the least squares matrices are invertible
    if diverged == 0
        % For each of the data collection (discrete time index)
        for k = 1:nbar
            % Initialize the optimal inputs to zero 
            uNew = [0; 0];
            % INNER LOOP
            for j = 1:(innerLoopMax-1)
                % Get the updated input value
                uLast = uNew;
                % Update the error model
                % Because of no anonymous functions we have modified f
                % fbar = @(e) A*e;
                % f = @(e) fbar(e)*tau + e;
                e_k_plus_1(:,k) = (A*e_vec(:,k)*tau) + e_vec(:,k) + g*uLast + h;
                % Compute the new optimal inputs
                % Partial derivative of rho with respect to e
                drhode = [1, 0, 0, 0;
                          0, 1, 0, 0;
                          0, 0, 1, 0;
                          0, 0, 0, 1;
                          2*e_vec(1,k), 0, 0, 0;
                          e_vec(2,k), e_vec(1,k), 0, 0;
                          e_vec(3,k), 0, e_vec(1,k), 0;
                          e_vec(4,k), 0, 0, e_vec(1,k);
                          0, 2*e_vec(2,k), 0, 0;
                          0, e_vec(3,k), e_vec(2,k), 0;
                          0, e_vec(4,k), 0, e_vec(2,k);
                          0, 0, 2*e_vec(3,k), 0;
                          0, 0, e_vec(4,k), e_vec(3,k);
                          0, 0, 0, 2*e_vec(4,k)];
                uNew  = -0.5*(R^(-1))*g'*drhode'*WcLast;
                
                % Check convergence of the optimal inputs
                if norm(uNew - uLast) < EpsilonPolicy
                    break;
                end
            end

            % Update the values for the least-squares computation
            % Critic neural network activation functions
            rhoE = [e_vec(1,k); e_vec(2,k); e_vec(3,k); e_vec(4,k);...
                    e_vec(1,k)^2; e_vec(1,k)*e_vec(2,k);...
                    e_vec(1,k)*e_vec(3,k); e_vec(1,k)*e_vec(4,k);...
                    e_vec(2,k)^2; e_vec(2,k)*e_vec(3,k);...
                    e_vec(2,k)*e_vec(4,k); e_vec(3,k)^2;...
                    e_vec(3,k)*e_vec(4,k); e_vec(4,k)^2];
           rhoEK = [e_k_plus_1(1,k); e_k_plus_1(2,k); e_k_plus_1(3,k);...
                    e_k_plus_1(4,k); e_k_plus_1(1,k)^2;...
                    e_k_plus_1(1,k)*e_k_plus_1(2,k);...
                    e_k_plus_1(1,k)*e_k_plus_1(3,k);...
                    e_k_plus_1(1,k)*e_k_plus_1(4,k);...
                    e_k_plus_1(2,k)^2; e_k_plus_1(2,k)*e_k_plus_1(3,k);...
                    e_k_plus_1(2,k)*e_k_plus_1(4,k); e_k_plus_1(3,k)^2;...
                    e_k_plus_1(3,k)*e_k_plus_1(4,k); e_k_plus_1(4,k)^2];
            % State penalizing function in the continuous cost function
            % Qbar = @(e) e'*Q_Mat*e; 
            % State penalizing function in the discretized cost function
            % Q = @(e) Qbar(e)*tau;
            V(k,:) = (e_vec(:,k)'*Q_Mat*e_vec(:,k)*tau) + uNew'*R*uNew + WcLast'*rhoEK;
            Lambda(k,:) = rhoE';
        end
    end

    % Verify the least square solution exists for the critic's weights
    % If the error data is consistent or there is no error, this will not
    % hold, so set the weights to what they were initially before the
    % simulation
    if det(Lambda'*Lambda) == 0
        weights = wcInit;
        break;
    end;

    % Calulcate least squares solution of critic's weights -- EQ 20
    WcNew = (Lambda'*Lambda)^(-1)*Lambda'*V;
    % Make sure the weights did not diverge
    % If the weights diverged, set the weights to what they were initially
    % before the simulation
    if isnan(WcNew)
        weights = wcInit;
        break;
    % Check for convergence of the critic weights
    elseif norm(WcNew - WcLast) < EpsilonWcritic               
        weights = WcNew;
        break;
    % If we reach the last iteration of the loop, just use the last weights
    elseif (i == (outerLoopMax-1))
        weights = WcNew;
    % If all else fails, just set the weights to the initial weights
    else
        weights = wcInit;
    end
    % If the weights did not converge, do another iteration of the loop
    WcLast = WcNew;
    end
    
    % Use the weights to determine the P matrix
    P_Mat = [weights(5) weights(6) weights(7) weights(8);
             weights(6) weights(9) weights(10) weights(11);
             weights(7) weights(10) weights(12) weights(13);
             weights(8) weights(11) weights(13) weights(14)];

    % Find the state-feedback gain EQ
    K = 0.5*(R_Mat^-1)*B'*P_Mat;
end
